simulink model "gm_optimized_area_multi_module_phase_shift_generator_built_in_counter"  (R2025b)
settings: Solver=FixedStepDiscrete  StartTime=0.0  StopTime=10e3  RelTol=1e-3
libraries: simulink x3, hdlmdlgenlib x1, hdlsllib x1
settings Model: Creator=KoayXianCong  LastModifiedBy=KoayXianCong
settings OptimizationCC: BlockReduction=off  ConditionallyExecuteInputs=off  DefaultParameterBehavior=Inlined  InheritOutputTypeSmallerThanSingle=on
settings DebuggingCC: ArtificialAlgebraicLoopMsg=error  InheritedTsInSrcMsg=none  SingleTaskRateTransMsg=error
settings HardwareCC: ProdBitPerPointer=32.0  ProdBitPerSizeT=32.0  ProdBitPerPtrDiffT=32.0  ProdLargestAtomicFloat=None  ProdIntDivRoundTo=Undefined  ProdEndianess=Unspecified  ProdWordSize=32.0  ProdHWDeviceType=ASIC/FPGA->ASIC/FPGA  TargetBitPerPointer=64.0  TargetBitPerSizeT=64.0  TargetBitPerPtrDiffT=64.0  TargetLongLongMode=on  TargetIntDivRoundTo=Zero  TargetEndianess=LittleEndian  TargetWordSize=64.0  TargetHWDeviceType=Custom Processor->MATLAB Host Computer  ProdEqTarget=off

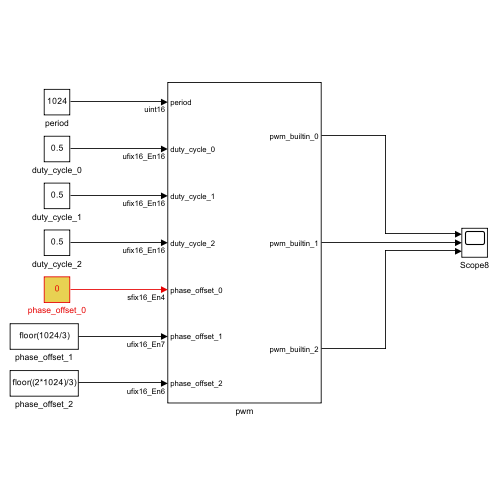
[thumbnail: Simulink's stored preview of the top-level diagram]
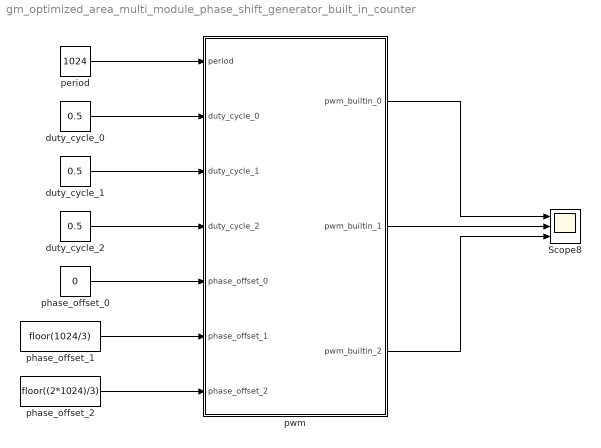
== system gm_optimized_area_multi_module_phase_shift_generator_built_in_counter ==
  Scope8 : Scope  NumInputPorts=3
      settings: ActiveDisplayYMinimum=-1  ActiveDisplayYMaximum=1  DataLoggingVariableName=ScopeData10  DataLoggingSaveFormat=Array
  duty_cycle_0 : Constant  Value=0.5  OutDataTypeStr=fixdt(0,16,16)
  duty_cycle_1 : Constant  Value=0.5  OutDataTypeStr=fixdt(0,16,16)
  duty_cycle_2 : Constant  Value=0.5  OutDataTypeStr=fixdt(0,16,16)
  period : Constant  Value=1024  OutDataTypeStr=uint16  SampleTime=1
  phase_offset_0 : Constant  Value=0  OutDataTypeStr=fixdt(1,16,4)
  phase_offset_1 : Constant  Value=floor(1024/3)  OutDataTypeStr=fixdt(0,16,7)
  phase_offset_2 : Constant  Value=floor((2*1024)/3)  OutDataTypeStr=fixdt(0,16,6)
  pwm : Subsystem
  wires:
  duty_cycle_2/1 -> pwm/4(duty_cycle_2)
  duty_cycle_1/1 -> pwm/3(duty_cycle_1)
  duty_cycle_0/1 -> pwm/2(duty_cycle_0)
  period/1 -> pwm/1(period)
  phase_offset_2/1 -> pwm/7(phase_offset_2)
  phase_offset_1/1 -> pwm/6(phase_offset_1)
  phase_offset_0/1 -> pwm/5(phase_offset_0)
  pwm/3(pwm_builtin_2) -> Scope8/3
  pwm/2(pwm_builtin_1) -> Scope8/2
  pwm/1(pwm_builtin_0) -> Scope8/1

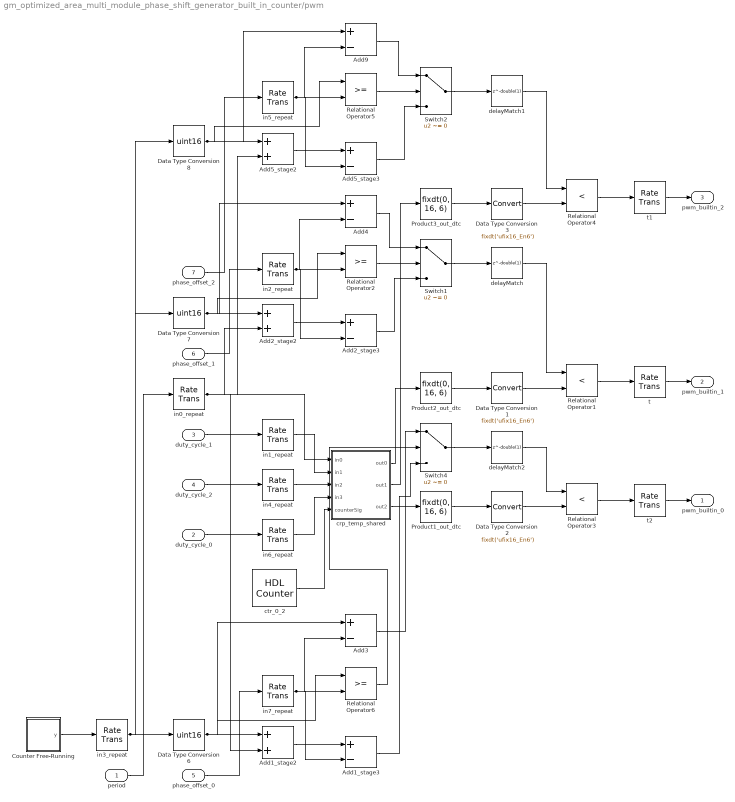
== system gm_optimized_area_multi_module_phase_shift_generator_built_in_counter/pwm ==
  period : Inport  OutDataTypeStr=uint16  PortDimensions=1  SampleTime=1
  duty_cycle_0 : Inport  Port=2  OutDataTypeStr=fixdt(0, 16, 16)  PortDimensions=1  SampleTime=1
  duty_cycle_1 : Inport  Port=3  OutDataTypeStr=fixdt(0, 16, 16)  PortDimensions=1  SampleTime=1
  duty_cycle_2 : Inport  Port=4  OutDataTypeStr=fixdt(0, 16, 16)  PortDimensions=1  SampleTime=1
  phase_offset_0 : Inport  Port=5  OutDataTypeStr=fixdt(1, 16, 4)  PortDimensions=1  SampleTime=1
  phase_offset_1 : Inport  Port=6  OutDataTypeStr=fixdt(0, 16, 7)  PortDimensions=1  SampleTime=1
  phase_offset_2 : Inport  Port=7  OutDataTypeStr=fixdt(0, 16, 6)  PortDimensions=1  SampleTime=1
  Add1_stage2 : Sum  OutDataTypeStr=fixdt(0, 17, 0)  AccumDataTypeStr=fixdt(1, 23, 4)  SampleTime=0.333333333333333
  Add1_stage3 : Sum  Inputs=+-  OutDataTypeStr=fixdt(1, 23, 4)  AccumDataTypeStr=fixdt(1, 23, 4)  SampleTime=0.333333333333333
  Add2_stage2 : Sum  OutDataTypeStr=fixdt(0, 17, 0)  AccumDataTypeStr=fixdt(1, 25, 7)  SampleTime=0.333333333333333
  Add2_stage3 : Sum  Inputs=+-  OutDataTypeStr=fixdt(1, 25, 7)  AccumDataTypeStr=fixdt(1, 25, 7)  SampleTime=0.333333333333333
  Add3 : Sum  Inputs=+-  OutDataTypeStr=fixdt(1, 22, 4)  AccumDataTypeStr=fixdt(1, 22, 4)  SampleTime=0.333333333333333
  Add4 : Sum  Inputs=+-  OutDataTypeStr=fixdt(1, 24, 7)  AccumDataTypeStr=fixdt(1, 24, 7)  SampleTime=0.333333333333333
  Add5_stage2 : Sum  OutDataTypeStr=fixdt(0, 17, 0)  AccumDataTypeStr=fixdt(1, 24, 6)  SampleTime=0.333333333333333
  Add5_stage3 : Sum  Inputs=+-  OutDataTypeStr=fixdt(1, 24, 6)  AccumDataTypeStr=fixdt(1, 24, 6)  SampleTime=0.333333333333333
  Add9 : Sum  Inputs=+-  OutDataTypeStr=fixdt(1, 23, 6)  AccumDataTypeStr=fixdt(1, 23, 6)  SampleTime=0.333333333333333
  Counter Free-Running : Subsystem  mask(Counter Free-Running){NumBits=double(10), tsamp=double(1)}
      mask prompts: NumBits "Simulink:masks:NumberOfBits_MP"; tsamp "Simulink:masks:SampleTime_MP"
      mask help: Simulink:masks:CounterFreeRunning_MD
  Data Type Conversion1 : DataTypeConversion  OutDataTypeStr=fixdt('ufix16_En6')
  Data Type Conversion2 : DataTypeConversion  OutDataTypeStr=fixdt('ufix16_En6')
  Data Type Conversion3 : DataTypeConversion  OutDataTypeStr=fixdt('ufix16_En6')
  Data Type Conversion6 : DataTypeConversion  OutDataTypeStr=uint16  SampleTime=0.333333333333333  SaturateOnIntegerOverflow=off  RndMeth=Floor
  Data Type Conversion7 : DataTypeConversion  OutDataTypeStr=uint16  SampleTime=0.333333333333333  SaturateOnIntegerOverflow=off  RndMeth=Floor
  Data Type Conversion8 : DataTypeConversion  OutDataTypeStr=uint16  SampleTime=0.333333333333333  SaturateOnIntegerOverflow=off  RndMeth=Floor
  Product1_out_dtc : DataTypeConversion  OutDataTypeStr=fixdt(0, 16, 6)  SampleTime=0.333333333333333  SaturateOnIntegerOverflow=off  RndMeth=Floor
  Product2_out_dtc : DataTypeConversion  OutDataTypeStr=fixdt(0, 16, 6)  SampleTime=0.333333333333333  SaturateOnIntegerOverflow=off  RndMeth=Floor
  Product3_out_dtc : DataTypeConversion  OutDataTypeStr=fixdt(0, 16, 6)  SampleTime=0.333333333333333  SaturateOnIntegerOverflow=off  RndMeth=Floor
  Relational Operator1 : RelationalOperator  Operator=<  OutDataTypeStr=boolean  SampleTime=0.333333333333333  InputSameDT=off
  Relational Operator2 : RelationalOperator  OutDataTypeStr=boolean  SampleTime=0.333333333333333  InputSameDT=off
  Relational Operator3 : RelationalOperator  Operator=<  OutDataTypeStr=boolean  SampleTime=0.333333333333333  InputSameDT=off
  Relational Operator4 : RelationalOperator  Operator=<  OutDataTypeStr=boolean  SampleTime=0.333333333333333  InputSameDT=off
  Relational Operator5 : RelationalOperator  OutDataTypeStr=boolean  SampleTime=0.333333333333333  InputSameDT=off
  Relational Operator6 : RelationalOperator  OutDataTypeStr=boolean  SampleTime=0.333333333333333  InputSameDT=off
  Switch1 : Switch  Criteria=u2 ~= 0  Threshold="fi(0,0,1,0,\"hex\",\"0\")"  OutDataTypeStr=fixdt(1, 25, 7)  SampleTime=0.333333333333333  SaturateOnIntegerOverflow=off  InputSameDT=off
  Switch2 : Switch  Criteria=u2 ~= 0  Threshold="fi(0,0,1,0,\"hex\",\"0\")"  OutDataTypeStr=fixdt(1, 24, 6)  SampleTime=0.333333333333333  SaturateOnIntegerOverflow=off  InputSameDT=off
  Switch4 : Switch  Criteria=u2 ~= 0  Threshold="fi(0,0,1,0,\"hex\",\"0\")"  OutDataTypeStr=fixdt(1, 23, 4)  SampleTime=0.333333333333333  SaturateOnIntegerOverflow=off  InputSameDT=off
  crp_temp_shared : Subsystem
  ctr_0_2 : hdlsllib/Sources/HDL Counter  CountType=Count limited  CountInit=double(0)  CountStep=double(1)  CountMax=double(2)  CountFromType=Initial value  CountFrom=double(0)  CountResetPort=off  CountLoadPort=off  CountEnbPort=off  CountDirPort=off  CountHitOutputPort=off  CountDataType=Unsigned  CountWordLen=2  CountFracLen=0  CountSampTime=0.333333333333333
  delayMatch : Delay  DelayLength=double(1)  InitialCondition=0  SampleTime=0.333333333333333
  delayMatch1 : Delay  DelayLength=double(1)  InitialCondition=0  SampleTime=0.333333333333333
  delayMatch2 : Delay  DelayLength=double(1)  InitialCondition=0  SampleTime=0.333333333333333
  in0_repeat : RateTransition  Integrity=off  Deterministic=off  OutPortSampleTimeOpt=Multiple of input port sample time  OutPortSampleTimeMultiple=1/3
  in1_repeat : RateTransition  Integrity=off  Deterministic=off  OutPortSampleTimeOpt=Multiple of input port sample time  OutPortSampleTimeMultiple=1/3
  in2_repeat : RateTransition  Integrity=off  Deterministic=off  OutPortSampleTimeOpt=Multiple of input port sample time  OutPortSampleTimeMultiple=1/3
  in3_repeat : RateTransition  Integrity=off  Deterministic=off  OutPortSampleTimeOpt=Multiple of input port sample time  OutPortSampleTimeMultiple=1/3
  in4_repeat : RateTransition  Integrity=off  Deterministic=off  OutPortSampleTimeOpt=Multiple of input port sample time  OutPortSampleTimeMultiple=1/3
  in5_repeat : RateTransition  Integrity=off  Deterministic=off  OutPortSampleTimeOpt=Multiple of input port sample time  OutPortSampleTimeMultiple=1/3
  in6_repeat : RateTransition  Integrity=off  Deterministic=off  OutPortSampleTimeOpt=Multiple of input port sample time  OutPortSampleTimeMultiple=1/3
  in7_repeat : RateTransition  Integrity=off  Deterministic=off  OutPortSampleTimeOpt=Multiple of input port sample time  OutPortSampleTimeMultiple=1/3
  t : RateTransition  InitialCondition=double(0)  OutPortSampleTimeOpt=Multiple of input port sample time  OutPortSampleTimeMultiple=3
  t1 : RateTransition  InitialCondition=double(0)  OutPortSampleTimeOpt=Multiple of input port sample time  OutPortSampleTimeMultiple=3
  t2 : RateTransition  InitialCondition=double(0)  OutPortSampleTimeOpt=Multiple of input port sample time  OutPortSampleTimeMultiple=3
  pwm_builtin_0 : Outport  SampleTime=1
  pwm_builtin_1 : Outport  Port=2  SampleTime=1
  pwm_builtin_2 : Outport  Port=3  SampleTime=1
  wires:
  t/1 -> pwm_builtin_1/1
  delayMatch/1 -> Relational Operator1/1
  Add2_stage3/1 -> Switch1/3
  Data Type Conversion6/1 -> Add3/1, Relational Operator6/1, Add1_stage2/1
  Data Type Conversion7/1 -> Add4/1, Relational Operator2/1, Add2_stage2/1
  Counter Free-Running/1(y) -> in3_repeat/1
  Add1_stage2/1 -> Add1_stage3/1
  in3_repeat/1 -> Data Type Conversion8/1, Data Type Conversion6/1, Data Type Conversion7/1
  phase_offset_2/1 -> in5_repeat/1
  delayMatch1/1 -> Relational Operator4/1
  Switch1/1 -> delayMatch/1
  period/1 -> in0_repeat/1
  Relational Operator2/1 -> Switch1/2
  Data Type Conversion8/1 -> Relational Operator5/1, Add5_stage2/1, Add9/1
  phase_offset_1/1 -> in2_repeat/1
  Product3_out_dtc/1 -> Data Type Conversion3/1
  in0_repeat/1 -> Add1_stage2/2, Add5_stage2/2, crp_temp_shared/1(in0), Add2_stage2/2
  duty_cycle_1/1 -> in1_repeat/1
  Add2_stage2/1 -> Add2_stage3/1
  duty_cycle_2/1 -> in4_repeat/1
  duty_cycle_0/1 -> in6_repeat/1
  Add4/1 -> Switch1/1
  phase_offset_0/1 -> in7_repeat/1
  Relational Operator6/1 -> Switch4/2
  in5_repeat/1 -> Add9/2, Add5_stage3/2, Relational Operator5/2
  Add5_stage2/1 -> Add5_stage3/1
  in2_repeat/1 -> Add2_stage3/2, Add4/2, Relational Operator2/2
  Product2_out_dtc/1 -> Data Type Conversion1/1
  in1_repeat/1 -> crp_temp_shared/2(in1)
  in4_repeat/1 -> crp_temp_shared/3(in2)
  Relational Operator3/1 -> t2/1
  in6_repeat/1 -> crp_temp_shared/4(in3)
  t1/1 -> pwm_builtin_2/1
  ctr_0_2/1 -> crp_temp_shared/5(counterSig)
  in7_repeat/1 -> Add1_stage3/2, Relational Operator6/2, Add3/2
  Add9/1 -> Switch2/1
  Relational Operator5/1 -> Switch2/2
  Add5_stage3/1 -> Switch2/3
  crp_temp_shared/1(out0) -> Product2_out_dtc/1
  Data Type Conversion1/1 -> Relational Operator1/2
  crp_temp_shared/2(out1) -> Product3_out_dtc/1
  crp_temp_shared/3(out2) -> Product1_out_dtc/1
  Add3/1 -> Switch4/1
  Add1_stage3/1 -> Switch4/3
  Switch2/1 -> delayMatch1/1
  Switch4/1 -> delayMatch2/1
  delayMatch2/1 -> Relational Operator3/1
  Product1_out_dtc/1 -> Data Type Conversion2/1
  Data Type Conversion3/1 -> Relational Operator4/2
  Data Type Conversion2/1 -> Relational Operator3/2
  Relational Operator4/1 -> t1/1
  Relational Operator1/1 -> t/1
  t2/1 -> pwm_builtin_0/1

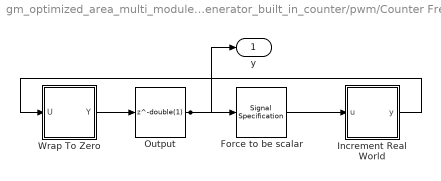
== system gm_optimized_area_multi_module_phase_shift_generator_built_in_counter/pwm/Counter Free-Running ==
  Force to be scalar : SignalSpecification  OutDataTypeStr=fixdt(0, 10, 0)  Dimensions=1
  Increment Real World : Subsystem  mask(Real World Value Increment){}
      mask help: Simulink:masks:RealWorldValueIncrement_MD
      mask Display: disp('V++')
  Output : Delay  DelayLength=double(1)  InitialCondition=0  SampleTime=1
  Wrap To Zero : Subsystem  mask(Wrap To Zero){Threshold=double(1023)}
      mask prompts: Threshold "Simulink:masks:Threshold_MP"
      mask help: Simulink:masks:WrapToZero_MD
  y : Outport  SampleTime=1
  wires:
  Increment Real World/1(y) -> Wrap To Zero/1(U)
  Wrap To Zero/1(Y) -> Output/1
  Output/1 -> Force to be scalar/1, y/1
  Force to be scalar/1 -> Increment Real World/1(u)

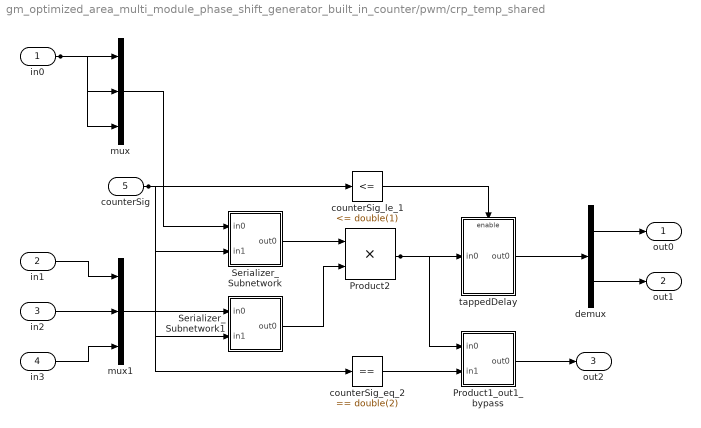
== system gm_optimized_area_multi_module_phase_shift_generator_built_in_counter/pwm/crp_temp_shared ==
  in0 : Inport  OutDataTypeStr=uint16  SampleTime=0.333333333333333
  in1 : Inport  Port=2  OutDataTypeStr=fixdt(0, 16, 16)  SampleTime=0.333333333333333
  in2 : Inport  Port=3  OutDataTypeStr=fixdt(0, 16, 16)  SampleTime=0.333333333333333
  in3 : Inport  Port=4  OutDataTypeStr=fixdt(0, 16, 16)  SampleTime=0.333333333333333
  counterSig : Inport  Port=5  OutDataTypeStr=fixdt(0, 2, 0)  SampleTime=0.333333333333333
  Product1_out1_bypass : Subsystem
  Product2 : Product  Inputs=**  OutDataTypeStr=fixdt(0, 32, 16)  SampleTime=0.333333333333333
  Serializer_Subnetwork : Subsystem
  Serializer_Subnetwork1 : Subsystem
  counterSig_eq_2 : simulink/Logic and Bit Operations/Compare To Constant  relop===  const=double(2)  OutDataTypeStr=boolean
  counterSig_le_1 : simulink/Logic and Bit Operations/Compare To Constant  relop=<=  const=double(1)  OutDataTypeStr=boolean
  demux : Demux  Outputs=2
  mux : Mux  Inputs=3
  mux1 : Mux  Inputs=3
  tappedDelay : Subsystem
  out0 : Outport  OutDataTypeStr=fixdt(0, 32, 16)  SampleTime=0.333333333333333
  out1 : Outport  Port=2  OutDataTypeStr=fixdt(0, 32, 16)  SampleTime=0.333333333333333
  out2 : Outport  Port=3  OutDataTypeStr=fixdt(0, 32, 16)  SampleTime=0.333333333333333
  wires:
  Serializer_Subnetwork/1(out0) -> Product2/1
  mux/1 -> Serializer_Subnetwork/1(in0)
  in0/1 -> mux/3, mux/2, mux/1
  in1/1 -> mux1/1
  in2/1 -> mux1/2
  in3/1 -> mux1/3
  counterSig/1 -> counterSig_eq_2/1, Serializer_Subnetwork1/2(in1), Serializer_Subnetwork/2(in1), counterSig_le_1/1
  mux1/1 -> Serializer_Subnetwork1/1(in0)
  Serializer_Subnetwork1/1(out0) -> Product2/2
  counterSig_le_1/1 -> tappedDelay/Enable
  Product2/1 -> tappedDelay/1(in0), Product1_out1_bypass/1(in0)
  counterSig_eq_2/1 -> Product1_out1_bypass/2(in1)
  tappedDelay/1(out0) -> demux/1
  Product1_out1_bypass/1(out0) -> out2/1
  demux/1 -> out0/1
  demux/2 -> out1/1

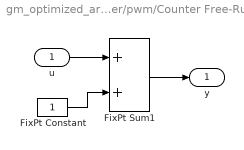
== system gm_optimized_area_multi_module_phase_shift_generator_built_in_counter/pwm/Counter Free-Running/Increment Real World ==
  u : Inport  OutDataTypeStr=fixdt(0, 10, 0)  SampleTime=1
  FixPt Constant : Constant  DisableCoverage=on  OutDataTypeStr=fixdt(0, 10, 0)  SampleTime=-1
  FixPt Sum1 : Sum  OutDataTypeStr=fixdt(0, 10, 0)  InputSameDT=on  LockScale=on
  y : Outport  SampleTime=1
  wires:
  u/1 -> FixPt Sum1/1
  FixPt Constant/1 -> FixPt Sum1/2
  FixPt Sum1/1 -> y/1

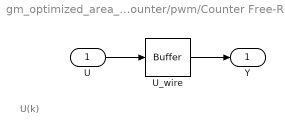
== system gm_optimized_area_multi_module_phase_shift_generator_built_in_counter/pwm/Counter Free-Running/Wrap To Zero ==
  note: U(k)
  U : Inport  OutDataTypeStr=fixdt(0, 10, 0)  SampleTime=1
  U_wire : hdlmdlgenlib/Buffer
  Y : Outport  SampleTime=1  InitialOutput=0
  wires:
  U/1 -> U_wire/1
  U_wire/1 -> Y/1

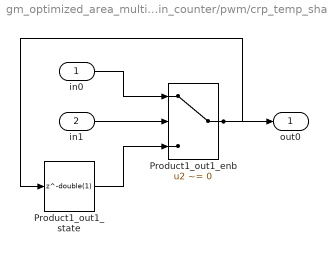
== system gm_optimized_area_multi_module_phase_shift_generator_built_in_counter/pwm/crp_temp_shared/Product1_out1_bypass ==
  in0 : Inport  OutDataTypeStr=fixdt(0, 32, 16)  SampleTime=0.333333333333333
  in1 : Inport  Port=2  OutDataTypeStr=boolean  SampleTime=0.333333333333333
  Product1_out1_enb : Switch  Criteria=u2 ~= 0  Threshold=double(0)  OutDataTypeStr=fixdt(0, 32, 16)  SampleTime=0.333333333333333  SaturateOnIntegerOverflow=off  InputSameDT=off
  Product1_out1_state : Delay  DelayLength=double(1)  InitialCondition=0  SampleTime=0.333333333333333
  out0 : Outport  OutDataTypeStr=fixdt(0, 32, 16)  SampleTime=0.333333333333333
  wires:
  in0/1 -> Product1_out1_enb/1
  Product1_out1_enb/1 -> Product1_out1_state/1, out0/1
  in1/1 -> Product1_out1_enb/2
  Product1_out1_state/1 -> Product1_out1_enb/3

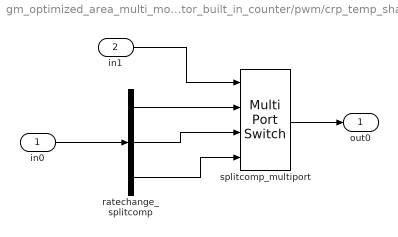
== system gm_optimized_area_multi_module_phase_shift_generator_built_in_counter/pwm/crp_temp_shared/Serializer_Subnetwork ==
  in0 : Inport  OutDataTypeStr=uint16  PortDimensions=[3]  SampleTime=0.333333333333333
  in1 : Inport  Port=2  OutDataTypeStr=fixdt(0, 2, 0)  SampleTime=0.333333333333333
  ratechange_splitcomp : Demux  Outputs=3
  splitcomp_multiport : MultiPortSwitch  DataPortOrder=Zero-based contiguous  DiagnosticForDefault=None  zeroidx=on  OutDataTypeStr=uint16  SampleTime=0.333333333333333  SaturateOnIntegerOverflow=off  InputSameDT=off
  out0 : Outport  OutDataTypeStr=uint16  SampleTime=0.333333333333333
  wires:
  in0/1 -> ratechange_splitcomp/1
  splitcomp_multiport/1 -> out0/1
  in1/1 -> splitcomp_multiport/1
  ratechange_splitcomp/2 -> splitcomp_multiport/3
  ratechange_splitcomp/1 -> splitcomp_multiport/2
  ratechange_splitcomp/3 -> splitcomp_multiport/4

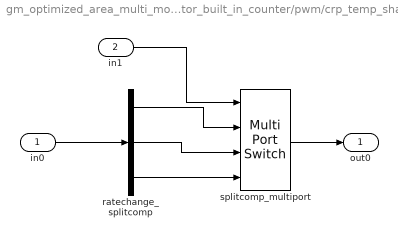
== system gm_optimized_area_multi_module_phase_shift_generator_built_in_counter/pwm/crp_temp_shared/Serializer_Subnetwork1 ==
  in0 : Inport  OutDataTypeStr=fixdt(0, 16, 16)  PortDimensions=[3]  SampleTime=0.333333333333333
  in1 : Inport  Port=2  OutDataTypeStr=fixdt(0, 2, 0)  SampleTime=0.333333333333333
  ratechange_splitcomp : Demux  Outputs=3
  splitcomp_multiport : MultiPortSwitch  DataPortOrder=Zero-based contiguous  DiagnosticForDefault=None  zeroidx=on  OutDataTypeStr=fixdt(0, 16, 16)  SampleTime=0.333333333333333  SaturateOnIntegerOverflow=off  InputSameDT=off
  out0 : Outport  OutDataTypeStr=fixdt(0, 16, 16)  SampleTime=0.333333333333333
  wires:
  in0/1 -> ratechange_splitcomp/1
  in1/1 -> splitcomp_multiport/1
  ratechange_splitcomp/1 -> splitcomp_multiport/2
  ratechange_splitcomp/3 -> splitcomp_multiport/4
  ratechange_splitcomp/2 -> splitcomp_multiport/3
  splitcomp_multiport/1 -> out0/1

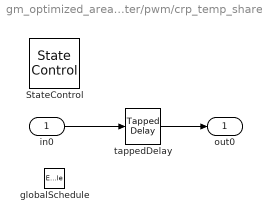
== system gm_optimized_area_multi_module_phase_shift_generator_built_in_counter/pwm/crp_temp_shared/tappedDelay ==
  in0 : Inport  OutDataTypeStr=fixdt(0, 32, 16)  SampleTime=0.333333333333333
  globalSchedule : EnablePort  OutDataTypeStr=boolean
  StateControl : StateControl  StateControl=Synchronous
  tappedDelay : simulink/Discrete/Tapped Delay  vinit=0  samptime=-1  NumDelays=double(2)  DelayOrder=Oldest  includeCurrent=off
  out0 : Outport  OutDataTypeStr=fixdt(0, 32, 16)  PortDimensions=[2]  SampleTime=0.333333333333333  InitialOutput=0
  wires:
  in0/1 -> tappedDelay/1
  tappedDelay/1 -> out0/1
